simulink model "gm_sampleModel1475_5_sub"  (R2023a)
settings: Solver=VariableStepAuto  StartTime=0.0  StopTime=10.0  RelTol=1e-3
settings Model: Creator=user1  LastModifiedBy=user1
settings OptimizationCC: BlockReduction=off  ConditionallyExecuteInputs=off
settings DebuggingCC: InheritedTsInSrcMsg=none

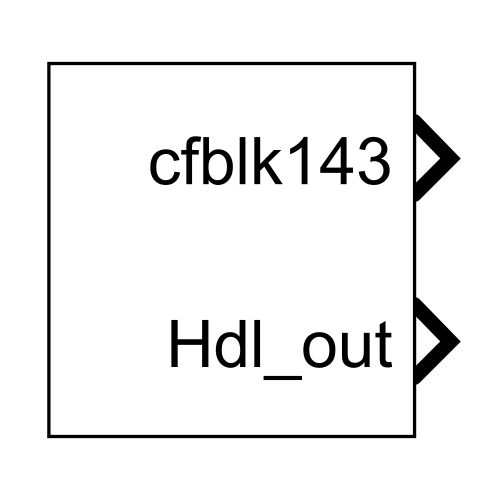
[thumbnail: Simulink's stored preview of the top-level diagram]
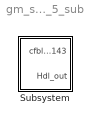
== system gm_sampleModel1475_5_sub ==
  Subsystem : Subsystem

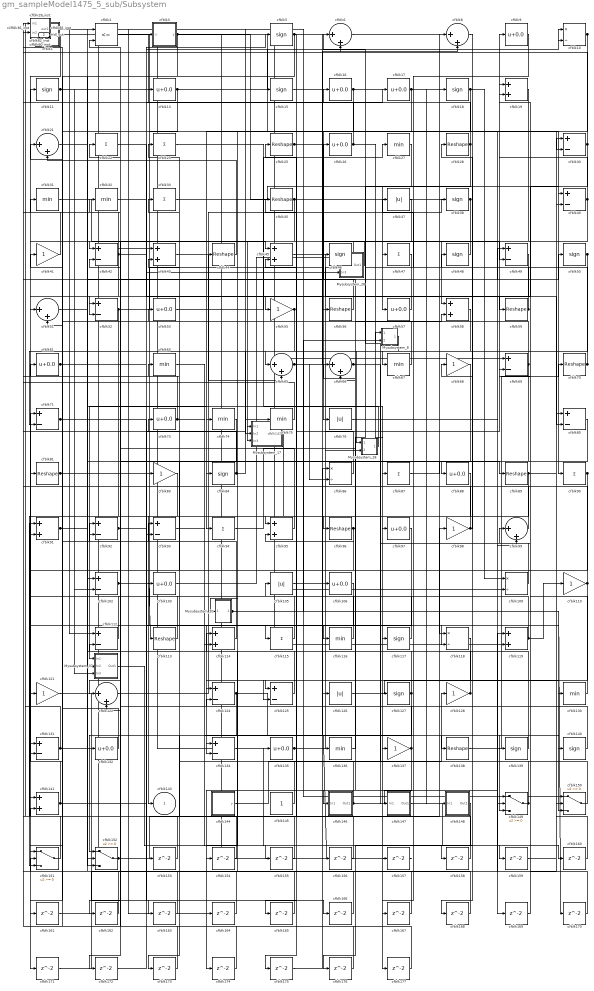
== system gm_sampleModel1475_5_sub/Subsystem ==
  Mysubsystem_17 : Subsystem
  Mysubsystem_18 : Subsystem
  Mysubsystem_20 : Subsystem
  Mysubsystem_28 : Subsystem
  Mysubsystem_37 : Subsystem
  Mysubsystem_8 : Subsystem
  cfblk1 : Subsystem  mask(Detect Rise Positive){vinit=double(0), InputProcessing=Elements as channels (sample based), OutDataTypeStr=uint8}
      mask prompts: vinit "Simulink:masks:InitialCondition_MP"; InputProcessing "Simulink:masks:InputProcessing_MP"; OutDataTypeStr "Simulink:masks:OutputDataType_MP"
      mask help: Simulink:masks:DetectRisePositive_MD
      mask init:
      | InputProcessing = 'Elements as channels (sample based)';
      | OutDataTypeStr = 'uint8';
      | vinit = double(0);
      mask TypeOptions InputProcessing: Simulink:masks:ColumnsAsChannelsFrameBased | Simulink:masks:ElementsAsChannelsSampleBased
      mask TypeOptions OutDataTypeStr: Simulink:masks:uint8 | Simulink:masks:boolean
      mask Display: fprintf('U > 0\n&  NOT\nU/z > 0')
  cfblk{10,86,109,118} (4 alike) : Product  Inputs=*/  OutDataTypeStr=uint8  RndMeth=Zero  SaturateOnIntegerOverflow=on
  cfblk{30,40,42,49,52,69,71,80,92..93,102,112,124..125,131,134} (16 alike) : Sum  Inputs=+-  OutDataTypeStr=uint8
  cfblk{9,13,16..17,26,53,57,61,73,88,97,103,106,132,135} (15 alike) : Bias  Bias=0.0  SaturateOnIntegerOverflow=off
  cfblk104_inst : Subsystem
  cfblk{37,76,105,126} (4 alike) : Abs  OutDataTypeStr=uint8  SaturateOnIntegerOverflow=off
  cfblk{5,11,15,18,38,46,48,50,84,117,127,139..140} (13 alike) : Signum
  cfblk{41,55,68,83,98,110,121,128,137} (9 alike) : Gain  OutDataTypeStr=uint8
  cfblk{25,28,35,44,56,59,70,81,89,96,113,138} (12 alike) : Reshape
  cfblk{19,43,45,58,91,95,114,119,141} (9 alike) : Sum  OutDataTypeStr=uint8
  cfblk{22..23,33,47,87,90,94,115} (8 alike) : Sum  Inputs=+  OutDataTypeStr=uint8
  cfblk{27,31..32,63,67,74..75,116,130,136} (10 alike) : MinMax  OutDataTypeStr=uint8
  cfblk120_inst : Subsystem
  cfblk{6,8,21,51,65..66,99,122} (8 alike) : Sum  Inputs=|++  OutDataTypeStr=uint8
  cfblk123_inst : Subsystem
  cfblk12_inst : Subsystem
  cfblk144 : Subsystem  mask(Counter Limited){uplimit=double(7), tsamp=double(-1)}
      mask prompts: uplimit "Simulink:masks:UpperLimit_MP"; tsamp "Simulink:masks:SampleTime_MP"
      mask help: Simulink:masks:CounterLimited_MD
      mask init:
      | nbits = double(8);
      | tsamp = double(-1);
      | uplimit = double(7);
  cfblk145 : Constant  OutDataTypeStr=uint8  SampleTime=-1
  cfblk146 : Subsystem
  cfblk147 : Subsystem
  cfblk148 : Subsystem
  cfblk{149..152} (4 alike) : Switch  OutDataTypeStr=uint8  SaturateOnIntegerOverflow=off  InputSameDT=off
  cfblk{153..177} (25 alike) : Delay  SampleTime=1
  cfblk2 : RelationalOperator  Operator=<=  OutDataTypeStr=boolean  InputSameDT=off
  cfblk24_inst : Subsystem
  cfblk29_inst : Subsystem
  cfblk3 : Subsystem  mask(Compare To Constant){relop=<=, const=double(3), OutDataTypeStr=uint8, ZeroCross=on}
      mask prompts: relop "Simulink:masks:Operator_MP"; const "Simulink:masks:ConstantValue_MP"; OutDataTypeStr "Simulink:masks:OutputDataType_MP"; ZeroCross "Simulink:masks:EnableZerocrossingDetection_MP"
      mask help: Simulink:masks:CompareToConstant_MD
      mask init:
      | OutDataTypeStr = 'uint8';
      | ZeroCross = 'on';
      | blkName = 'sampleModel1475_5_sub/Subsystem/cfblk3';
      | const = double(3);
      | const_str = '3.0';
      | const_val = double(3);
      | relop = '<=';
      | setValue = 'fixdt(0, 8)';
      | str = '<= 3';
      mask TypeOptions relop: == | ~= | < | <= | >= | >
      mask TypeOptions OutDataTypeStr: Simulink:masks:uint8 | Simulink:masks:boolean
      mask Callback ZeroCross: sl('zeroCrossEnable', gcbh);
      mask Display: disp(str)
  cfblk36_inst : Subsystem
  cfblk60_inst : Subsystem
  cfblk82_inst : Subsystem
  cfblk85_inst : Subsystem
  cfblk143 : Outport  OutDataTypeStr=uint8  SampleTime=1  VectorParamsAs1DForOutWhenUnconnected=off
  Hdl_out : Outport  Port=2  OutDataTypeStr=uint8  SampleTime=1
  wires:
  Mysubsystem_17/1(cfblk143) -> cfblk143/1
  Mysubsystem_18/1(Out1) -> Mysubsystem_37/1(In1)
  Mysubsystem_20/1(Out1) -> cfblk170/1, Mysubsystem_8/2(In2), Mysubsystem_28/2(In2)
  Mysubsystem_28/1(Out1) -> cfblk171/1
  Mysubsystem_37/1(Out1) -> cfblk155/1
  Mysubsystem_8/1(Out1) -> Mysubsystem_17/3(In3)
  cfblk1/1(Y) -> cfblk141/1
  cfblk10/1 -> cfblk76/1, cfblk67/1
  cfblk102/1 -> cfblk113/1, cfblk177/1
  cfblk103/1 -> Mysubsystem_28/1(In1)
  cfblk104_inst/1(out1) -> cfblk8/1
  cfblk105/1 -> cfblk9/1
  cfblk106/1 -> cfblk134/2
  cfblk109/1 -> Mysubsystem_8/1(In1)
  cfblk11/1 -> cfblk150/3, cfblk102/2
  cfblk110/1 -> cfblk71/1, cfblk137/1
  cfblk112/1 -> cfblk61/1
  cfblk113/1 -> cfblk31/1
  cfblk114/1 -> cfblk41/1
  cfblk115/1 -> cfblk92/1
  cfblk116/1 -> cfblk81/1
  cfblk117/1 -> cfblk105/1
  cfblk118/1 -> cfblk134/1
  cfblk119/1 -> cfblk25/1, cfblk110/1
  cfblk12_inst/1(out1) -> cfblk150/1
  cfblk120_inst/1(out1) -> cfblk69/1
  cfblk121/1 -> cfblk163/1
  cfblk122/1 -> cfblk38/1
  cfblk123_inst/1(out1) -> cfblk135/1
  cfblk124/1 -> cfblk152/1, cfblk149/3, cfblk149/1
  cfblk125/1 -> cfblk23/1
  cfblk126/1 -> cfblk130/1
  cfblk127/1 -> cfblk92/2, cfblk26/1, cfblk173/1
  cfblk128/1 -> cfblk43/2, cfblk125/1
  cfblk13/1 -> cfblk161/1, cfblk10/1, cfblk90/1
  cfblk130/1 -> cfblk19/1
  cfblk131/1 -> cfblk36_inst/1(in1), cfblk132/1
  cfblk132/1 -> cfblk11/1
  cfblk134/1 -> cfblk160/1
  cfblk135/1 -> cfblk156/1, Mysubsystem_18/2(In2)
  cfblk136/1 -> cfblk66/1
  cfblk137/1 -> cfblk2/2, cfblk174/1
  cfblk138/1 -> cfblk70/1
  cfblk139/1 -> cfblk102/1
  cfblk140/1 -> cfblk6/1
  cfblk141/1 -> cfblk91/2, Mysubsystem_28/3(In3)
  cfblk144/1(y) -> cfblk128/1
  cfblk145/1 -> cfblk63/1
  cfblk146/1(Out1) -> cfblk73/1, cfblk149/2
  cfblk147/1(Out1) -> cfblk159/1
  cfblk148/1(Out1) -> cfblk176/1
  cfblk149/1 -> cfblk16/1, cfblk33/1
  cfblk15/1 -> cfblk118/2
  cfblk150/1 -> cfblk114/1
  cfblk151/1 -> cfblk24_inst/2(in2)
  cfblk152/1 -> cfblk98/1, cfblk22/1
  cfblk153/1 -> cfblk141/2
  cfblk154/1 -> cfblk93/1
  cfblk155/1 -> cfblk91/1
  cfblk156/1 -> cfblk36_inst/2(in2)
  cfblk157/1 -> cfblk1/1(U)
  cfblk158/1 -> cfblk45/2
  cfblk159/1 -> cfblk30/1
  cfblk16/1 -> cfblk126/1, cfblk106/1, cfblk94/1
  cfblk160/1 -> cfblk150/2
  cfblk161/1 -> cfblk119/1
  cfblk162/1 -> cfblk60_inst/2(in2)
  cfblk163/1 -> cfblk2/1
  cfblk164/1 -> cfblk151/2
  cfblk165/1 -> cfblk131/1
  cfblk166/1 -> cfblk124/2
  cfblk167/1 -> cfblk12_inst/2(in2)
  cfblk168/1 -> cfblk29_inst/1(in1)
  cfblk169/1 -> cfblk99/1
  cfblk17/1 -> cfblk175/1, cfblk148/1(In1)
  cfblk170/1 -> cfblk69/2
  cfblk171/1 -> cfblk80/1
  cfblk172/1 -> cfblk10/2
  cfblk173/1 -> cfblk112/2
  cfblk174/1 -> cfblk82_inst/2(in2)
  cfblk175/1 -> cfblk86/1
  cfblk176/1 -> cfblk42/2
  cfblk177/1 -> cfblk51/2
  cfblk18/1 -> cfblk127/1, cfblk124/1, cfblk109/1
  cfblk19/1 -> cfblk168/1
  cfblk2/1 -> cfblk30/2
  cfblk21/1 -> cfblk84/1
  cfblk22/1 -> cfblk55/1
  cfblk23/1 -> cfblk117/1
  cfblk24_inst/1(out1) -> cfblk164/1, cfblk109/2
  cfblk25/1 -> cfblk8/2, cfblk49/2
  cfblk26/1 -> cfblk3/1(u), cfblk87/1
  cfblk27/1 -> cfblk57/1
  cfblk28/1 -> cfblk104_inst/2(in2), cfblk136/1
  cfblk29_inst/1(out1) -> cfblk18/1
  cfblk3/1(y) -> cfblk152/3, cfblk169/1
  cfblk30/1 -> cfblk85_inst/2(in2), cfblk85_inst/1(in1), cfblk59/1
  cfblk31/1 -> cfblk45/1
  cfblk32/1 -> cfblk56/1
  cfblk33/1 -> cfblk40/1
  cfblk35/1 -> cfblk42/1, cfblk122/2
  cfblk36_inst/1(out1) -> cfblk82_inst/1(in1), cfblk43/1
  cfblk37/1 -> Mysubsystem_17/1(In1)
  cfblk38/1 -> cfblk58/1, Hdl_out/1
  cfblk40/1 -> cfblk52/2, cfblk19/2
  cfblk41/1 -> cfblk60_inst/1(in1)
  cfblk42/1 -> cfblk21/1, cfblk17/1, cfblk152/2
  cfblk43/1 -> cfblk65/2
  cfblk44/1 -> cfblk21/2
  cfblk45/1 -> cfblk80/2
  cfblk46/1 -> cfblk44/1
  cfblk47/1 -> cfblk151/1
  cfblk48/1 -> cfblk47/1
  cfblk49/1 -> cfblk65/1
  cfblk5/1 -> cfblk95/1, cfblk51/1, cfblk138/1
  cfblk50/1 -> cfblk125/2, Mysubsystem_18/1(In1)
  cfblk51/1 -> cfblk74/1
  cfblk52/1 -> cfblk6/2, cfblk151/3
  cfblk53/1 -> cfblk27/1
  cfblk55/1 -> cfblk71/2, Mysubsystem_17/2(In2)
  cfblk56/1 -> cfblk123_inst/2(in2)
  cfblk57/1 -> cfblk52/1
  cfblk58/1 -> cfblk165/1
  cfblk59/1 -> cfblk28/1, cfblk123_inst/1(in1)
  cfblk6/1 -> cfblk118/1
  cfblk60_inst/1(out1) -> cfblk119/2
  cfblk61/1 -> cfblk5/1, cfblk49/1
  cfblk63/1 -> cfblk114/2
  cfblk65/1 -> cfblk46/1, cfblk86/2
  cfblk66/1 -> cfblk140/1, cfblk147/1(In1)
  cfblk67/1 -> cfblk53/1
  cfblk68/1 -> cfblk122/1
  cfblk69/1 -> cfblk12_inst/1(in1), cfblk103/1
  cfblk70/1 -> cfblk37/1, cfblk120_inst/2(in2)
  cfblk71/1 -> cfblk88/1, cfblk115/1
  cfblk73/1 -> cfblk120_inst/1(in1), cfblk157/1
  cfblk74/1 -> cfblk93/2
  cfblk75/1 -> cfblk104_inst/1(in1)
  cfblk76/1 -> cfblk99/2
  cfblk8/1 -> cfblk158/1
  cfblk80/1 -> cfblk96/1
  cfblk81/1 -> cfblk83/1, cfblk166/1
  cfblk82_inst/1(out1) -> cfblk112/1, cfblk153/1
  cfblk83/1 -> Mysubsystem_37/2(In2)
  cfblk84/1 -> cfblk24_inst/1(in1), cfblk15/1
  cfblk85_inst/1(out1) -> cfblk13/1
  cfblk86/1 -> cfblk35/1
  cfblk87/1 -> cfblk89/1
  cfblk88/1 -> cfblk167/1
  cfblk89/1 -> cfblk40/2, cfblk172/1, Mysubsystem_20/1(In1)
  cfblk9/1 -> cfblk97/1
  cfblk90/1 -> cfblk162/1, cfblk121/1
  cfblk91/1 -> cfblk50/1, Mysubsystem_37/3(In3)
  cfblk92/1 -> cfblk116/1, cfblk75/1
  cfblk93/1 -> cfblk139/1
  cfblk94/1 -> cfblk58/2
  cfblk95/1 -> cfblk32/1
  cfblk96/1 -> cfblk95/2, cfblk154/1, cfblk146/1(In1)
  cfblk97/1 -> cfblk131/2
  cfblk98/1 -> cfblk66/2, cfblk48/1, cfblk68/1
  cfblk99/1 -> cfblk29_inst/2(in2)

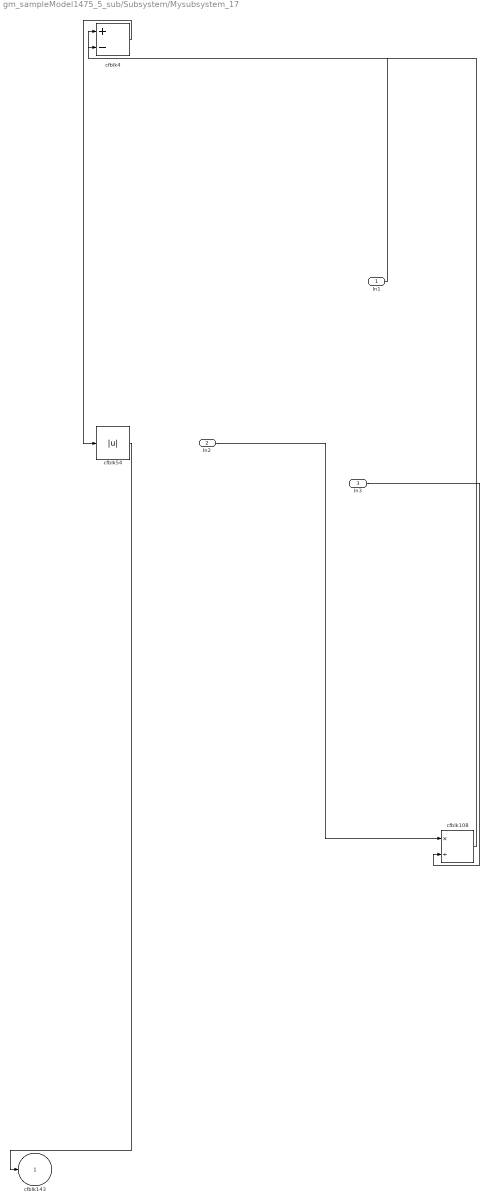
== system gm_sampleModel1475_5_sub/Subsystem/Mysubsystem_17 ==
  In1 : Inport  OutDataTypeStr=uint8  PortDimensions=1  SampleTime=1
  In2 : Inport  Port=2  OutDataTypeStr=uint8  PortDimensions=1  SampleTime=1
  In3 : Inport  Port=3  OutDataTypeStr=uint8  PortDimensions=1  SampleTime=1
  cfblk108 : Product  Inputs=*/  RndMeth=Zero  SaturateOnIntegerOverflow=on
  cfblk4 : Sum  Inputs=+-
  cfblk54 : Abs  SaturateOnIntegerOverflow=off
  cfblk143 : Outport  SampleTime=1  VectorParamsAs1DForOutWhenUnconnected=off
  wires:
  In1/1 -> cfblk4/1
  In2/1 -> cfblk108/1
  In3/1 -> cfblk108/2
  cfblk108/1 -> cfblk4/2
  cfblk4/1 -> cfblk54/1
  cfblk54/1 -> cfblk143/1

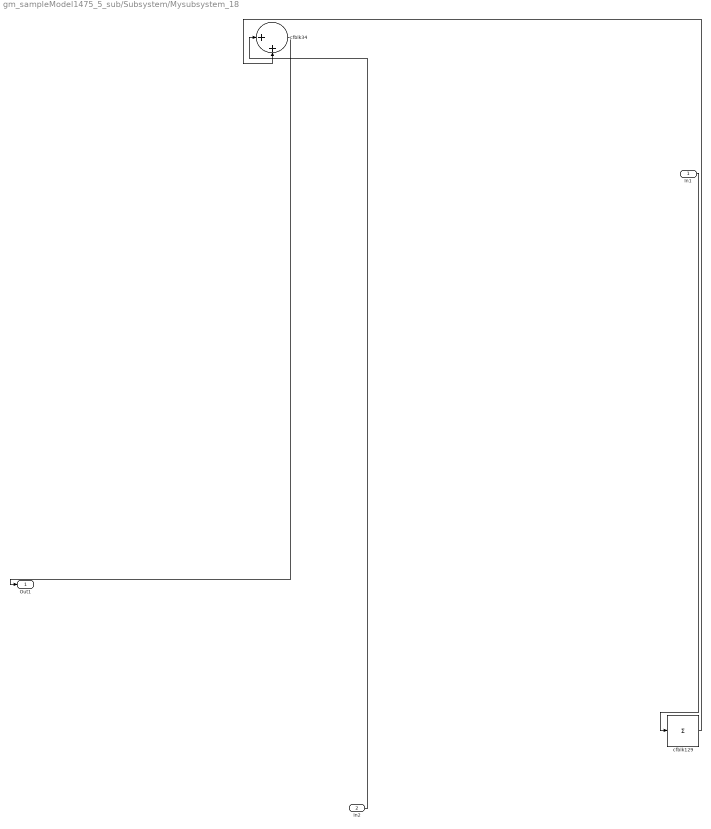
== system gm_sampleModel1475_5_sub/Subsystem/Mysubsystem_18 ==
  In1 : Inport  OutDataTypeStr=uint8  PortDimensions=1  SampleTime=1
  In2 : Inport  Port=2  OutDataTypeStr=uint8  PortDimensions=1  SampleTime=1
  cfblk129 : Sum  Inputs=+
  cfblk34 : Sum  Inputs=|++
  Out1 : Outport  SampleTime=1
  wires:
  In1/1 -> cfblk129/1
  In2/1 -> cfblk34/1
  cfblk129/1 -> cfblk34/2
  cfblk34/1 -> Out1/1

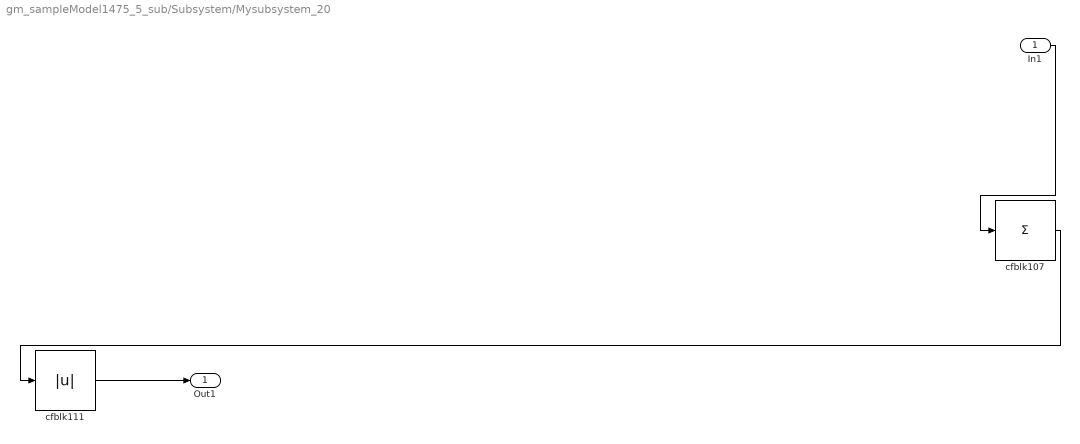
== system gm_sampleModel1475_5_sub/Subsystem/Mysubsystem_20 ==
  In1 : Inport  OutDataTypeStr=uint8  PortDimensions=1  SampleTime=1
  cfblk107 : Sum  Inputs=+
  cfblk111 : Abs  SaturateOnIntegerOverflow=off
  Out1 : Outport  SampleTime=1
  wires:
  In1/1 -> cfblk107/1
  cfblk107/1 -> cfblk111/1
  cfblk111/1 -> Out1/1

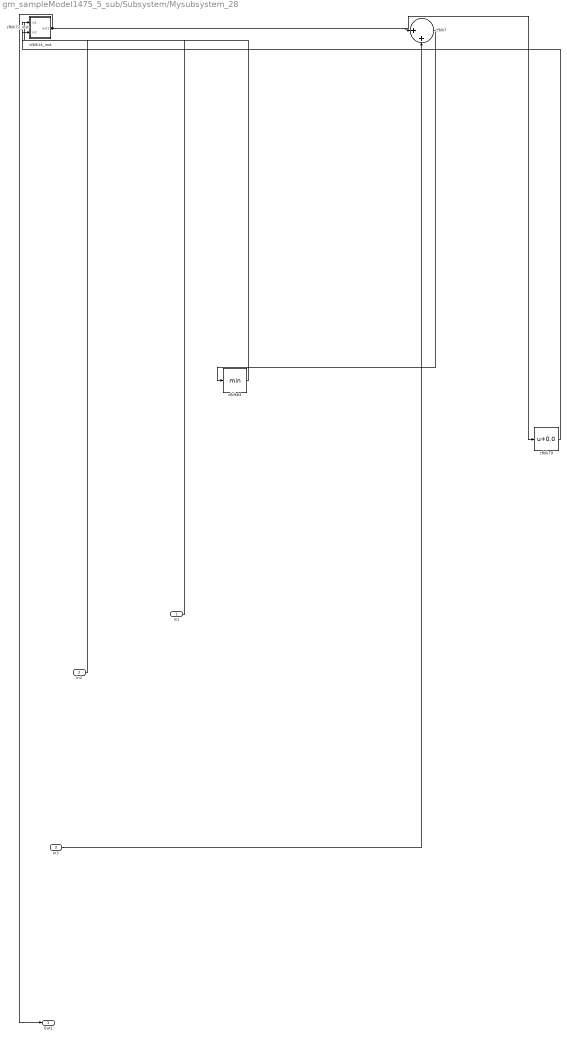
== system gm_sampleModel1475_5_sub/Subsystem/Mysubsystem_28 ==
  In1 : Inport  OutDataTypeStr=uint8  PortDimensions=1  SampleTime=1
  In2 : Inport  Port=2  OutDataTypeStr=uint8  PortDimensions=1  SampleTime=1
  In3 : Inport  Port=3  OutDataTypeStr=uint8  PortDimensions=1  SampleTime=1
  cfblk14_inst : Subsystem
  cfblk64 : MinMax
  cfblk7 : Sum  Inputs=|++
  cfblk77_inst : Subsystem
  cfblk79 : Bias  Bias=0.0  SaturateOnIntegerOverflow=off
  Out1 : Outport  SampleTime=1
  wires:
  In1/1 -> cfblk14_inst/1(in1)
  In2/1 -> cfblk14_inst/2(in2)
  In3/1 -> cfblk7/2
  cfblk14_inst/1(out1) -> cfblk79/1, cfblk7/1
  cfblk64/1 -> cfblk77_inst/1(in1)
  cfblk7/1 -> cfblk64/1
  cfblk77_inst/1(out1) -> Out1/1
  cfblk79/1 -> cfblk77_inst/2(in2)

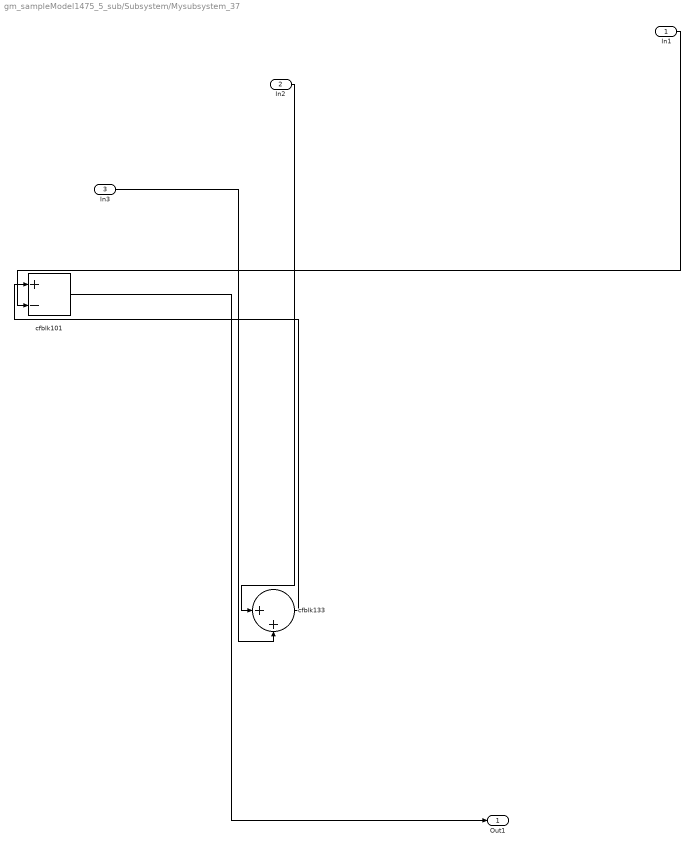
== system gm_sampleModel1475_5_sub/Subsystem/Mysubsystem_37 ==
  In1 : Inport  OutDataTypeStr=uint8  PortDimensions=1  SampleTime=1
  In2 : Inport  Port=2  OutDataTypeStr=uint8  PortDimensions=1  SampleTime=1
  In3 : Inport  Port=3  OutDataTypeStr=uint8  PortDimensions=1  SampleTime=1
  cfblk101 : Sum  Inputs=+-
  cfblk133 : Sum  Inputs=|++
  Out1 : Outport  SampleTime=1
  wires:
  In1/1 -> cfblk101/2
  In2/1 -> cfblk133/1
  In3/1 -> cfblk133/2
  cfblk101/1 -> Out1/1
  cfblk133/1 -> cfblk101/1

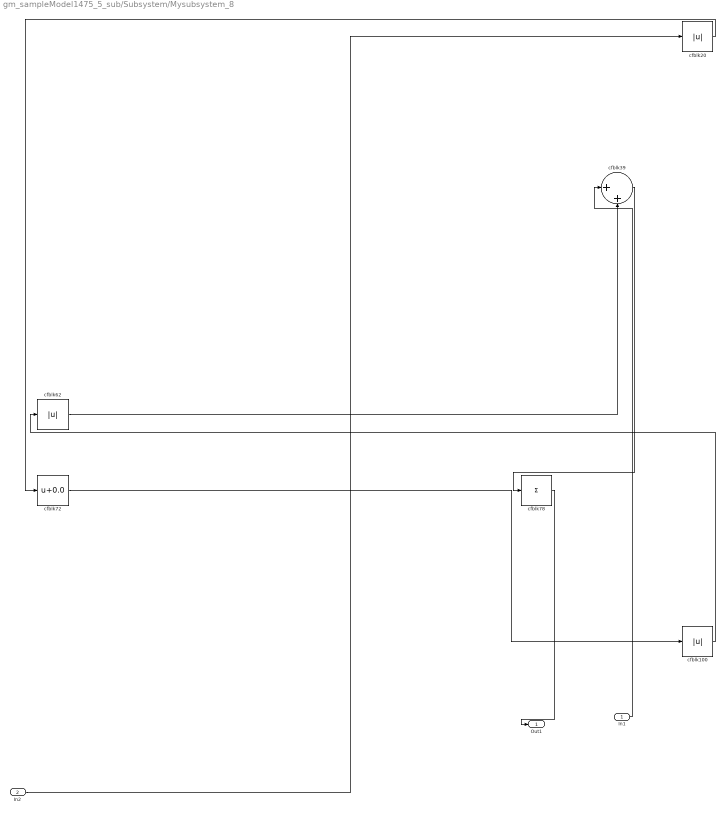
== system gm_sampleModel1475_5_sub/Subsystem/Mysubsystem_8 ==
  In1 : Inport  OutDataTypeStr=uint8  PortDimensions=1  SampleTime=1
  In2 : Inport  Port=2  OutDataTypeStr=uint8  PortDimensions=1  SampleTime=1
  cfblk100 : Abs  SaturateOnIntegerOverflow=off
  cfblk20 : Abs  SaturateOnIntegerOverflow=off
  cfblk39 : Sum  Inputs=|++
  cfblk62 : Abs  SaturateOnIntegerOverflow=off
  cfblk72 : Bias  Bias=0.0  SaturateOnIntegerOverflow=off
  cfblk78 : Sum  Inputs=+
  Out1 : Outport  SampleTime=1
  wires:
  In1/1 -> cfblk39/1
  In2/1 -> cfblk20/1
  cfblk100/1 -> cfblk62/1
  cfblk20/1 -> cfblk72/1
  cfblk39/1 -> cfblk78/1
  cfblk62/1 -> cfblk39/2
  cfblk72/1 -> cfblk100/1
  cfblk78/1 -> Out1/1

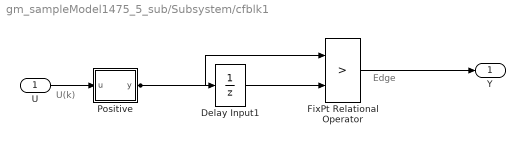
== system gm_sampleModel1475_5_sub/Subsystem/cfblk1 ==
  note: U(k)
  note: Edge
  U : Inport  OutDataTypeStr=uint8  SampleTime=1
  Delay Input1 : UnitDelay  Description=Store in Global RAM  DisableCoverage=on  InitialCondition=vinit  SampleTime=-1  HasFrameUpgradeWarning=on
  FixPt Relational Operator : RelationalOperator  Operator=>  OutDataTypeStr=fixdt(0, 8)  ZeroCross=off  InputSameDT=off
  Positive : Subsystem  mask(Compare To Zero){relop=>, OutDataTypeStr=boolean, ZeroCross=off}
      mask prompts: relop "Simulink:masks:Operator_MP"; OutDataTypeStr "Simulink:masks:OutputDataType_MP"; ZeroCross "Simulink:masks:EnableZerocrossingDetection_MP"
      mask help: Simulink:masks:CompareToZero_MD
      mask init:
      | OutDataTypeStr = 'boolean';
      | ZeroCross = 'off';
      | blkName = 'sampleModel1475_5_sub/Subsystem/cfblk1/Positive';
      | relop = '>';
      | setValue = 'boolean';
      mask TypeOptions relop: == | ~= | < | <= | >= | >
      mask TypeOptions OutDataTypeStr: Simulink:masks:uint8 | Simulink:masks:boolean
      mask Callback ZeroCross: sl('zeroCrossEnable', gcbh);
      mask Display: disp([relop,' 0'])
  Y : Outport  SampleTime=1
  wires:
  U/1 -> Positive/1(u)
  Delay Input1/1 -> FixPt Relational Operator/2
  FixPt Relational Operator/1 -> Y/1
  Positive/1(y) -> FixPt Relational Operator/1, Delay Input1/1

== system gm_sampleModel1475_5_sub/Subsystem/cfblk104_inst ==
  in1 : Inport  OutDataTypeStr=uint8  SampleTime=1
  in2 : Inport  Port=2  OutDataTypeStr=uint8  SampleTime=1
  mul_cfblk104_dotp_mulcomp : Product  Inputs=**  OutDataTypeStr=uint8  SampleTime=1
  out1 : Outport  OutDataTypeStr=uint8  SampleTime=1
  wires:
  in1/1 -> mul_cfblk104_dotp_mulcomp/1
  in2/1 -> mul_cfblk104_dotp_mulcomp/2
  mul_cfblk104_dotp_mulcomp/1 -> out1/1

== system gm_sampleModel1475_5_sub/Subsystem/cfblk120_inst ==
  in1 : Inport  OutDataTypeStr=uint8  SampleTime=1
  in2 : Inport  Port=2  OutDataTypeStr=uint8  SampleTime=1
  mul_cfblk120_dotp_mulcomp : Product  Inputs=**  OutDataTypeStr=uint8  SampleTime=1
  out1 : Outport  OutDataTypeStr=uint8  SampleTime=1
  wires:
  in1/1 -> mul_cfblk120_dotp_mulcomp/1
  in2/1 -> mul_cfblk120_dotp_mulcomp/2
  mul_cfblk120_dotp_mulcomp/1 -> out1/1

== system gm_sampleModel1475_5_sub/Subsystem/cfblk123_inst ==
  in1 : Inport  OutDataTypeStr=uint8  SampleTime=1
  in2 : Inport  Port=2  OutDataTypeStr=uint8  SampleTime=1
  mul_cfblk123_dotp_mulcomp : Product  Inputs=**  OutDataTypeStr=uint8  SampleTime=1
  out1 : Outport  OutDataTypeStr=uint8  SampleTime=1
  wires:
  in1/1 -> mul_cfblk123_dotp_mulcomp/1
  in2/1 -> mul_cfblk123_dotp_mulcomp/2
  mul_cfblk123_dotp_mulcomp/1 -> out1/1

== system gm_sampleModel1475_5_sub/Subsystem/cfblk12_inst ==
  in1 : Inport  OutDataTypeStr=uint8  SampleTime=1
  in2 : Inport  Port=2  OutDataTypeStr=uint8  SampleTime=1
  mul_cfblk12_dotp_mulcomp : Product  Inputs=**  OutDataTypeStr=uint8  SampleTime=1
  out1 : Outport  OutDataTypeStr=uint8  SampleTime=1
  wires:
  in1/1 -> mul_cfblk12_dotp_mulcomp/1
  in2/1 -> mul_cfblk12_dotp_mulcomp/2
  mul_cfblk12_dotp_mulcomp/1 -> out1/1

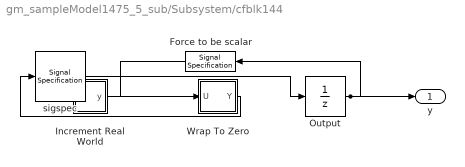
== system gm_sampleModel1475_5_sub/Subsystem/cfblk144 ==
  Force to be scalar : SignalSpecification  DisableCoverage=on  Dimensions=1
  Increment Real World : Subsystem  mask(Real World Value Increment){}
      mask help: Simulink:masks:RealWorldValueIncrement_MD
      mask Display: disp('V++')
  Output : UnitDelay  InitialCondition=0.0  SampleTime=tsamp  HasFrameUpgradeWarning=on
  Wrap To Zero : Subsystem  mask(Wrap To Zero){Threshold=double(7)}
      mask prompts: Threshold "Simulink:masks:Threshold_MP"
      mask help: Simulink:masks:WrapToZero_MD
  sigspec : SignalSpecification  OutDataTypeStr=uint8  Dimensions=1
  y : Outport  SampleTime=1
  wires:
  Force to be scalar/1 -> Increment Real World/1(u)
  Increment Real World/1(y) -> Wrap To Zero/1(U)
  Output/1 -> Force to be scalar/1, y/1
  Wrap To Zero/1(Y) -> sigspec/1
  sigspec/1 -> Output/1

== system gm_sampleModel1475_5_sub/Subsystem/cfblk146 ==
  In1 : Inport  OutDataTypeStr=uint8  PortDimensions=1  SampleTime=1
  Out1 : Outport  SampleTime=1
  wires:
  In1/1 -> Out1/1

== system gm_sampleModel1475_5_sub/Subsystem/cfblk147 ==
  In1 : Inport  OutDataTypeStr=uint8  PortDimensions=1  SampleTime=1
  Out1 : Outport  SampleTime=1
  wires:
  In1/1 -> Out1/1

== system gm_sampleModel1475_5_sub/Subsystem/cfblk148 ==
  In1 : Inport  OutDataTypeStr=uint8  PortDimensions=1  SampleTime=1
  Out1 : Outport  SampleTime=1
  wires:
  In1/1 -> Out1/1

== system gm_sampleModel1475_5_sub/Subsystem/cfblk24_inst ==
  in1 : Inport  OutDataTypeStr=uint8  SampleTime=1
  in2 : Inport  Port=2  OutDataTypeStr=uint8  SampleTime=1
  mul_cfblk24_dotp_mulcomp : Product  Inputs=**  OutDataTypeStr=uint8  SampleTime=1
  out1 : Outport  OutDataTypeStr=uint8  SampleTime=1
  wires:
  in1/1 -> mul_cfblk24_dotp_mulcomp/1
  in2/1 -> mul_cfblk24_dotp_mulcomp/2
  mul_cfblk24_dotp_mulcomp/1 -> out1/1

== system gm_sampleModel1475_5_sub/Subsystem/cfblk29_inst ==
  in1 : Inport  OutDataTypeStr=uint8  SampleTime=1
  in2 : Inport  Port=2  OutDataTypeStr=uint8  SampleTime=1
  mul_cfblk29_dotp_mulcomp : Product  Inputs=**  OutDataTypeStr=uint8  SampleTime=1
  out1 : Outport  OutDataTypeStr=uint8  SampleTime=1
  wires:
  in1/1 -> mul_cfblk29_dotp_mulcomp/1
  in2/1 -> mul_cfblk29_dotp_mulcomp/2
  mul_cfblk29_dotp_mulcomp/1 -> out1/1

== system gm_sampleModel1475_5_sub/Subsystem/cfblk3 ==
  u : Inport  OutDataTypeStr=uint8  SampleTime=1
  Compare : RelationalOperator  Operator=<=  OutDataTypeStr=fixdt(0, 8)
  Constant : Constant  DisableCoverage=on  Value=const  OutDataTypeStr=Inherit: Inherit via back propagation  SampleTime=-1
  y : Outport  SampleTime=1
  wires:
  u/1 -> Compare/1
  Compare/1 -> y/1
  Constant/1 -> Compare/2

== system gm_sampleModel1475_5_sub/Subsystem/cfblk36_inst ==
  in1 : Inport  OutDataTypeStr=uint8  SampleTime=1
  in2 : Inport  Port=2  OutDataTypeStr=uint8  SampleTime=1
  mul_cfblk36_dotp_mulcomp : Product  Inputs=**  OutDataTypeStr=uint8  SampleTime=1
  out1 : Outport  OutDataTypeStr=uint8  SampleTime=1
  wires:
  in1/1 -> mul_cfblk36_dotp_mulcomp/1
  in2/1 -> mul_cfblk36_dotp_mulcomp/2
  mul_cfblk36_dotp_mulcomp/1 -> out1/1

== system gm_sampleModel1475_5_sub/Subsystem/cfblk60_inst ==
  in1 : Inport  OutDataTypeStr=uint8  SampleTime=1
  in2 : Inport  Port=2  OutDataTypeStr=uint8  SampleTime=1
  mul_cfblk60_dotp_mulcomp : Product  Inputs=**  OutDataTypeStr=uint8  SampleTime=1
  out1 : Outport  OutDataTypeStr=uint8  SampleTime=1
  wires:
  in1/1 -> mul_cfblk60_dotp_mulcomp/1
  in2/1 -> mul_cfblk60_dotp_mulcomp/2
  mul_cfblk60_dotp_mulcomp/1 -> out1/1

== system gm_sampleModel1475_5_sub/Subsystem/cfblk82_inst ==
  in1 : Inport  OutDataTypeStr=uint8  SampleTime=1
  in2 : Inport  Port=2  OutDataTypeStr=uint8  SampleTime=1
  mul_cfblk82_dotp_mulcomp : Product  Inputs=**  OutDataTypeStr=uint8  SampleTime=1
  out1 : Outport  OutDataTypeStr=uint8  SampleTime=1
  wires:
  in1/1 -> mul_cfblk82_dotp_mulcomp/1
  in2/1 -> mul_cfblk82_dotp_mulcomp/2
  mul_cfblk82_dotp_mulcomp/1 -> out1/1

== system gm_sampleModel1475_5_sub/Subsystem/cfblk85_inst ==
  in1 : Inport  OutDataTypeStr=uint8  SampleTime=1
  in2 : Inport  Port=2  OutDataTypeStr=uint8  SampleTime=1
  mul_cfblk85_dotp_mulcomp : Product  Inputs=**  OutDataTypeStr=uint8  SampleTime=1
  out1 : Outport  OutDataTypeStr=uint8  SampleTime=1
  wires:
  in1/1 -> mul_cfblk85_dotp_mulcomp/1
  in2/1 -> mul_cfblk85_dotp_mulcomp/2
  mul_cfblk85_dotp_mulcomp/1 -> out1/1

== system gm_sampleModel1475_5_sub/Subsystem/Mysubsystem_28/cfblk14_inst ==
  in1 : Inport  OutDataTypeStr=uint8  SampleTime=1
  in2 : Inport  Port=2  OutDataTypeStr=uint8  SampleTime=1
  mul_cfblk14_dotp_mulcomp : Product  Inputs=**  OutDataTypeStr=uint16  SampleTime=1
  out1 : Outport  OutDataTypeStr=uint16  SampleTime=1
  wires:
  in1/1 -> mul_cfblk14_dotp_mulcomp/1
  in2/1 -> mul_cfblk14_dotp_mulcomp/2
  mul_cfblk14_dotp_mulcomp/1 -> out1/1

== system gm_sampleModel1475_5_sub/Subsystem/Mysubsystem_28/cfblk77_inst ==
  in1 : Inport  OutDataTypeStr=uint16  SampleTime=1
  in2 : Inport  Port=2  OutDataTypeStr=uint16  SampleTime=1
  mul_cfblk77_dotp_mulcomp : Product  Inputs=**  OutDataTypeStr=uint32  SampleTime=1
  out1 : Outport  OutDataTypeStr=uint32  SampleTime=1
  wires:
  in1/1 -> mul_cfblk77_dotp_mulcomp/1
  in2/1 -> mul_cfblk77_dotp_mulcomp/2
  mul_cfblk77_dotp_mulcomp/1 -> out1/1

== system gm_sampleModel1475_5_sub/Subsystem/cfblk1/Positive ==
  u : Inport  OutDataTypeStr=uint8  SampleTime=1
  Compare : RelationalOperator  Operator=>  OutDataTypeStr=boolean  ZeroCross=off
  Constant : Constant  DisableCoverage=on  Value=0  OutDataTypeStr=Inherit: Inherit via back propagation  SampleTime=-1  PreserveConstantTs=on
  y : Outport  SampleTime=1
  wires:
  u/1 -> Compare/1
  Compare/1 -> y/1
  Constant/1 -> Compare/2

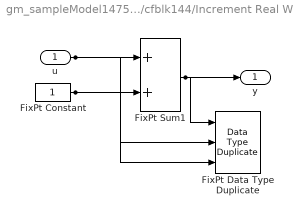
== system gm_sampleModel1475_5_sub/Subsystem/cfblk144/Increment Real World ==
  u : Inport  OutDataTypeStr=uint8  SampleTime=1
  FixPt Constant : Constant  DisableCoverage=on  OutDataTypeStr=Inherit: Inherit via back propagation  SampleTime=-1
  FixPt Data Type Duplicate : DataTypeDuplicate  DisableCoverage=on  NumInputPorts=3
  FixPt Sum1 : Sum  InputSameDT=on  OutDataTypeStr=Inherit: Inherit via back propagation  LockScale=on
  y : Outport  SampleTime=1
  wires:
  u/1 -> FixPt Sum1/1, FixPt Data Type Duplicate/2
  FixPt Constant/1 -> FixPt Sum1/2, FixPt Data Type Duplicate/3
  FixPt Sum1/1 -> FixPt Data Type Duplicate/1, y/1

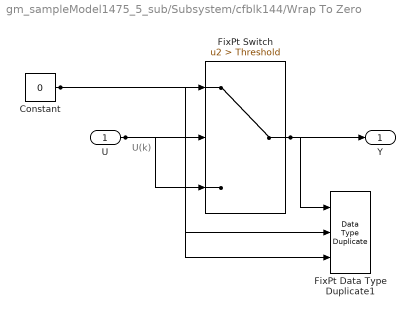
== system gm_sampleModel1475_5_sub/Subsystem/cfblk144/Wrap To Zero ==
  note: U(k)
  U : Inport  OutDataTypeStr=uint8  SampleTime=1
  Constant : Constant  DisableCoverage=on  Value=0  OutDataTypeStr=Inherit: Inherit via back propagation  SampleTime=-1
  FixPt Data Type Duplicate1 : DataTypeDuplicate  DisableCoverage=on  NumInputPorts=3
  FixPt Switch : Switch  Criteria=u2 > Threshold  Threshold=Threshold  OutDataTypeStr=Inherit: Inherit via back propagation  ZeroCross=off  SaturateOnIntegerOverflow=off  InputSameDT=off
  Y : Outport  SampleTime=1
  wires:
  U/1 -> FixPt Switch/3, FixPt Switch/2, FixPt Data Type Duplicate1/2
  Constant/1 -> FixPt Switch/1, FixPt Data Type Duplicate1/3
  FixPt Switch/1 -> FixPt Data Type Duplicate1/1, Y/1
